simulink model "MassSpringDamper_Model"  (R2019b)
settings: Solver=VariableStepAuto  StartTime=0.0  StopTime=10.0  RelTol=1e-3
values from neighbouring files (symbols this model uses):
  A = MSD_2.A    [ComputerLab04.m]
  B = MSD_2.B    [ComputerLab04.m]
  C = MSD_2.C    [ComputerLab04.m]
  D = MSD_1.D    [ComputerLab04.m]
settings Model: Creator=james  LastModifiedBy=james
settings DataIOCC: SaveOutput=off  SignalLogging=off  DSMLogging=off

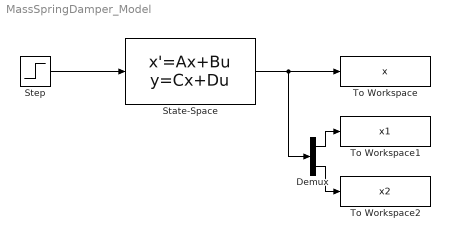
== system MassSpringDamper_Model ==
  Demux : Demux  Outputs=2
  State-Space : StateSpace  A=A  B=B  C=C  D=D  InitialCondition=0
  Step : Step  SampleTime=0
  To Workspace : ToWorkspace  VariableName=x  SampleTime=-1
  To Workspace1 : ToWorkspace  VariableName=x1  SampleTime=-1
  To Workspace2 : ToWorkspace  VariableName=x2  SampleTime=-1
  wires:
  Step/1 -> State-Space/1
  State-Space/1 -> Demux/1, To Workspace/1
  Demux/2 -> To Workspace2/1
  Demux/1 -> To Workspace1/1
